simulink model "FOC_PMSM_Developing"  (R2023b)
settings: Solver=VariableStepAuto  StartTime=0.0  StopTime=10.0  RelTol=1e-3
values from neighbouring files (symbols this model uses):
  B = 11e-5    (= 0.00011)    [FOC_For_PMSM.m]    (also in FOC_For_PMSM_Parameters.m)
  J = 0.47e-4    (= 4.7e-05)    [FOC_For_PMSM.m]    (also in FOC_For_PMSM_Parameters.m)
  Ld = 7e-2    (= 0.07)    [FOC_For_PMSM.m]    (also in FOC_For_PMSM_Parameters.m)
  Lq = 7e-2    (= 0.07)    [FOC_For_PMSM.m]    (also in FOC_For_PMSM_Parameters.m)
  p = 2    [FOC_For_PMSM.m]    (also in FOC_For_PMSM_Parameters.m)
  Rs = 2.98    [FOC_For_PMSM.m]    (also in FOC_For_PMSM_Parameters.m)
libraries: spsDCVoltageSourceLib x1, spsdq0toabcLib x1, spsPermanentMagnetSynchronousMachineLib x1, spsUniversalBridgeLib x1, spspowerguiLib x1
settings Model: Creator=hkurt  LastModifiedBy=hkurt

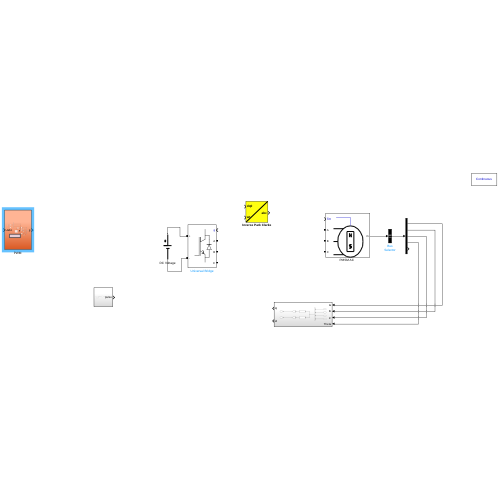
[thumbnail: Simulink's stored preview of the top-level diagram]
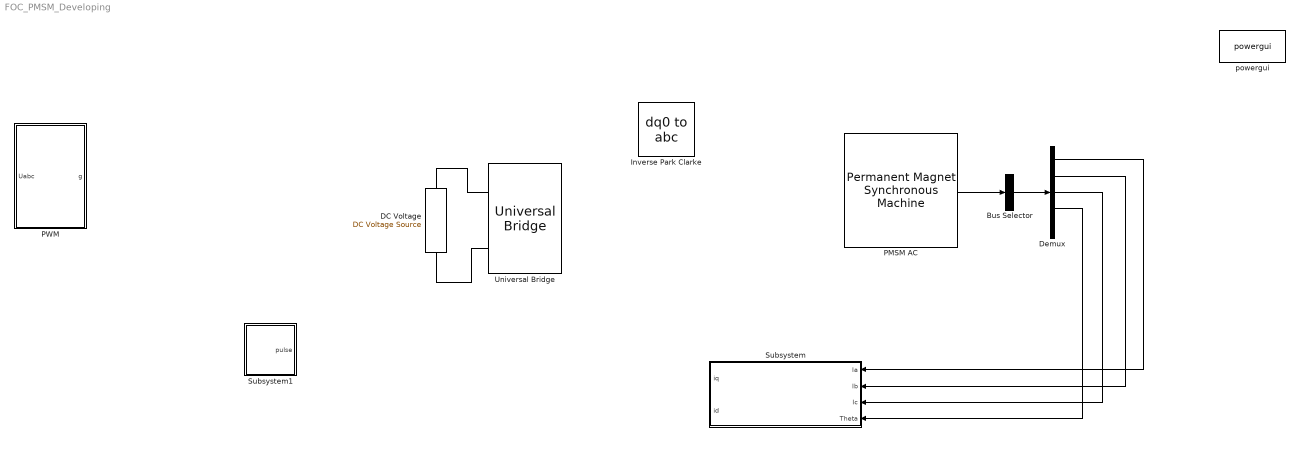
== system FOC_PMSM_Developing ==
  Bus Selector : BusSelector  OutputSignals=Stator current is_a (A),Stator current is_b (A),Stator current is_c (A),Rotor angle thetam (rad),Rotor speed wm (rad/s)  OutputAsBus=on
  DC Voltage : spsDCVoltageSourceLib/DC Voltage Source  Amplitude=600  Measurements=None
  Demux : Demux  Outputs=5
  Inverse Park Clarke : spsdq0toabcLib/dq0 to abc  Alignment=Aligned with phase A axis
  "PMSM AC  " : spsPermanentMagnetSynchronousMachineLib/Permanent Magnet Synchronous Machine  NbPhases=3  FluxDistribution=Sinusoidal  RotorType=Salient-pole  MechanicalLoad=Torque Tm  PresetModel=No  ShowDetailedParameters=on  MeasurementBus=off  Resistance=Rs  Inductance=8.5e-3  dqInductances=[Ld, Lq]  La=0.000395  MachineConstant=Flux linkage established by magnets (V.s)  Flux=flux  VoltageCst=45.345  TorqueCst=0.375  Flat=120  Mechanical=[J B p 0]  PolePairs=4  InitialConditions=[0,0, 0,0]  InitialConditions5ph=[0 0 0 0 0 0]  RefAngle=90 degrees behind phase A axis (modified Park)  IterativeDiscreteModel=Trapezoidal non iterative  TsBlock=-1  TsPowergui=0
  "PWM " : Subsystem
  Subsystem : Subsystem
  Subsystem1 : Subsystem
  Universal Bridge : spsUniversalBridgeLib/Universal Bridge  Arms=3  SnubberResistance=1e5  SnubberCapacitance=inf  Device=IGBT / Diodes  Ron=1e-3  Lon=0  ForwardVoltages="[  0  0  ]"  ForwardVoltage=0  GTOparameters=[ 10e-6 , 20e-6 ]  IGBTparameters=[ 1e-6 , 2e-6 ]  Measurements=None  Measurements_2=None  converterType=Rectifier
  powergui : spspowerguiLib/powergui  Priority=1  SimulationMode=Continuous  SampleTime=50e-6  frequency=60  Iterations=50  frequencyindice=60  Pbase=100e6  ErrMax=1e-4  UnitsV=kV  UnitsW=MW  buscounter=0  FunctionMessages=off  echomessages=off  EnableUseOfTLC=off  CurrentSourceSwitches=off  DisableSnubberDevices=off  DisableRonSwitches=off  DisableVfSwitches=off  DisplayEquations=off  AutomaticDiscreteSolvers=off  SolverType=Tustin/Backward Euler (TBE)  Interpol=off  ExternalGateDelay=off  methode=off  Ts=100  x0status=blocks  SPID=on  SwTol=0  HookPort=off  NonlinearTolerance=1e-4  nMaxIteration=100  ContinueOnMaxIteration=off  RestoreLinks=warning  ResistiveCurrentMeasurement=off  Frange=[0:2:500]  Ylog=off  Xlog=on  ShowGrid=off  save=off  variable=ZData  structure=0  ZoomFFT=off  StartTime=0.0  cycles=1  DisplayStyle=1  fundamental=60  FreqAxis=off  MaxFrequency=1000  frequencyindicesteady=1  RmsSteady=1  display=off
  wires:
  "PMSM AC  "/1 -> Bus Selector/1
  Bus Selector/1 -> Demux/1
  Demux/1 -> Subsystem/1(Ia)
  Demux/2 -> Subsystem/2(Ib)
  Demux/3 -> Subsystem/3(Ic)
  Demux/4 -> Subsystem/4(Theta)
  connections:
  DC Voltage/RConn1 -- Universal Bridge/RConn1
  DC Voltage/LConn1 -- Universal Bridge/RConn2

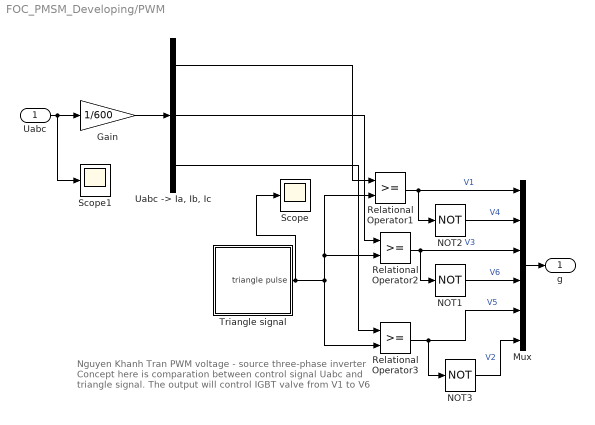
== system FOC_PMSM_Developing/PWM  ==
  note: Nguyen Khanh Tran
      | PWM voltage - source three-phase inverter
      | Concept here is comparation between
      | control signal Uabc and triangle signal.
      | The output will control IGBT valve from V1 to V6
  Uabc : Inport
  Gain : Gain  Gain=1/600
  Mux : Mux  Inputs=6
  NOT1 : Logic  Operator=NOT  IconShape=distinctive  AllPortsSameDT=off  OutDataTypeStr=boolean
  NOT2 : Logic  Operator=NOT  IconShape=distinctive  AllPortsSameDT=off  OutDataTypeStr=boolean
  NOT3 : Logic  Operator=NOT  IconShape=distinctive  AllPortsSameDT=off  OutDataTypeStr=boolean
  Relational Operator1 : RelationalOperator  OutDataTypeStr=boolean  RndMeth=Simplest  InputSameDT=off
  Relational Operator2 : RelationalOperator  OutDataTypeStr=boolean  RndMeth=Simplest  InputSameDT=off
  Relational Operator3 : RelationalOperator  OutDataTypeStr=boolean  RndMeth=Simplest  InputSameDT=off
  Scope : Scope
  Scope1 : Scope
  "Triangle signal " : Subsystem
  "Uabc -> Ia, Ib, Ic " : Demux  Outputs=3
  g : Outport
  wires:
  NOT1/1 -> Mux/4  "V6"
  "Uabc -> Ia, Ib, Ic "/2 -> Relational Operator2/1
  "Uabc -> Ia, Ib, Ic "/1 -> Relational Operator1/1
  "Uabc -> Ia, Ib, Ic "/3 -> Relational Operator3/1
  Relational Operator2/1 -> NOT1/1, Mux/3  "V3"
  Relational Operator1/1 -> NOT2/1, Mux/1  "V1"
  "Triangle signal "/1(triangle pulse) -> Relational Operator2/2, Relational Operator1/2, Relational Operator3/2, Scope/1
  Relational Operator3/1 -> NOT3/1, Mux/5  "V5"
  NOT3/1 -> Mux/6  "V2"
  NOT2/1 -> Mux/2  "V4"
  Mux/1 -> g/1
  Uabc/1 -> Scope1/1, Gain/1
  Gain/1 -> "Uabc -> Ia, Ib, Ic "/1

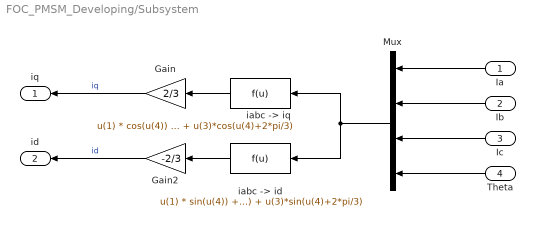
== system FOC_PMSM_Developing/Subsystem ==
  Ia : Inport
  Ib : Inport  Port=2
  Ic : Inport  Port=3
  Theta : Inport  Port=4
  Gain : Gain  Gain=2/3
  Gain2 : Gain  Gain=-2/3
  Mux : Mux
  "iabc -> id" : Fcn  Expr=u(1) * sin(u(4)) + u(2) *sin(u(4) - 2*pi/3) + u(3)*sin(u(4)+2*pi/3)
  "iabc -> iq" : Fcn  Expr=u(1) * cos(u(4)) + u(2) *cos(u(4) - 2*pi/3) + u(3)*cos(u(4)+2*pi/3)
  iq : Outport
  id : Outport  Port=2
  wires:
  Gain2/1 -> id/1  "id"
  Gain/1 -> iq/1  "iq"
  "iabc -> id"/1 -> Gain2/1
  "iabc -> iq"/1 -> Gain/1
  Mux/1 -> "iabc -> iq"/1, "iabc -> id"/1
  Ia/1 -> Mux/1
  Ib/1 -> Mux/2
  Ic/1 -> Mux/3
  Theta/1 -> Mux/4

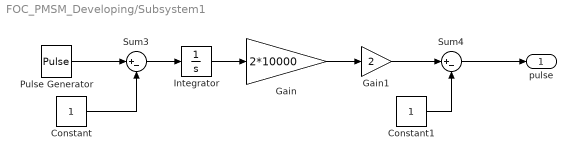
== system FOC_PMSM_Developing/Subsystem1 ==
  Constant : Constant
  Constant1 : Constant
  Gain : Gain  Gain=2*10000
  Gain1 : Gain  Gain=2
  Integrator : Integrator
  Pulse Generator : DiscretePulseGenerator  PulseType=Time based  Amplitude=2  Period=1/10000  PulseWidth=50
  Sum3 : Sum  Inputs=|+-
  Sum4 : Sum  Inputs=|+-
  pulse : Outport
  wires:
  Integrator/1 -> Gain/1
  Sum4/1 -> pulse/1
  Sum3/1 -> Integrator/1
  Gain/1 -> Gain1/1
  Constant1/1 -> Sum4/2
  Constant/1 -> Sum3/2
  Gain1/1 -> Sum4/1
  Pulse Generator/1 -> Sum3/1

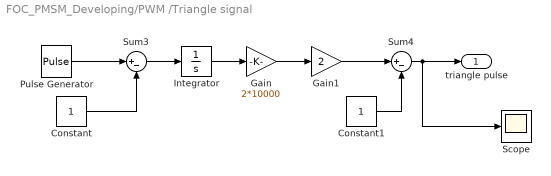
== system FOC_PMSM_Developing/PWM /Triangle signal  ==
  Constant : Constant
  Constant1 : Constant
  Gain : Gain  Gain=2*10000
  Gain1 : Gain  Gain=2
  Integrator : Integrator
  Pulse Generator : DiscretePulseGenerator  PulseType=Time based  Amplitude=2  Period=1/10000  PulseWidth=50
  Scope : Scope
  Sum3 : Sum  Inputs=|+-
  Sum4 : Sum  Inputs=|+-
  triangle pulse : Outport
  wires:
  Integrator/1 -> Gain/1
  Gain/1 -> Gain1/1
  Constant1/1 -> Sum4/2
  Gain1/1 -> Sum4/1
  Pulse Generator/1 -> Sum3/1
  Sum3/1 -> Integrator/1
  Constant/1 -> Sum3/2
  Sum4/1 -> Scope/1, triangle pulse/1
